simulink model "Mojtaba_simulink"  (R2022b)
settings: Solver=FixedStepAuto  StartTime=0.0  StopTime=5  FixedStep=1e-3  RelTol=1e-3
values from neighbouring files (symbols this model uses):
  Mojtaba_hand = Hand('Mojtaba_hand')    [create_Hand_Model_wt_Muscles.m]    (also in create_MSK_Mojtaba.m)
settings Model: Creator=ge26jow  LastModifiedBy=ge26jow

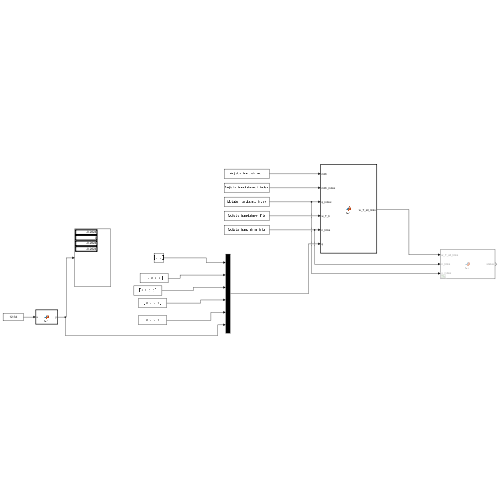
[thumbnail: Simulink's stored preview of the top-level diagram]
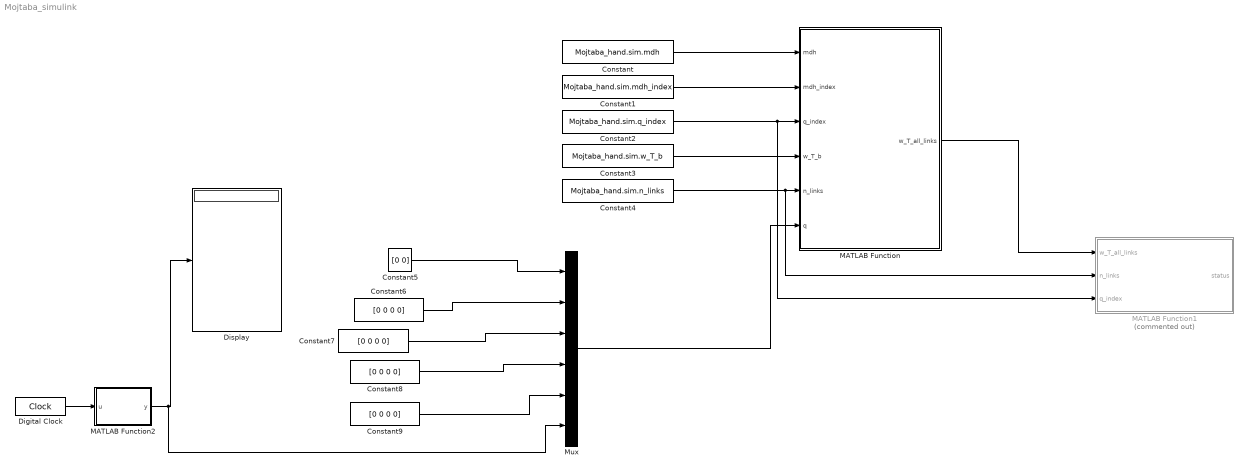
== system Mojtaba_simulink ==
  Constant : Constant  Value=Mojtaba_hand.sim.mdh
  Constant1 : Constant  Value=Mojtaba_hand.sim.mdh_index
  Constant2 : Constant  Value=Mojtaba_hand.sim.q_index
  Constant3 : Constant  Value=Mojtaba_hand.sim.w_T_b
  Constant4 : Constant  Value=Mojtaba_hand.sim.n_links
  Constant5 : Constant  Value=[0 0]
  Constant{6..9} (4 alike) : Constant  Value=[0 0 0 0]
  Digital Clock : DigitalClock  SampleTime=1e-2
  Display : Display
  MATLAB Function : MATLAB Function  TreatAsAtomicUnit=on
  MATLAB Function1 : MATLAB Function  Commented=on  TreatAsAtomicUnit=on
  MATLAB Function2 : MATLAB Function  TreatAsAtomicUnit=on
  Mux : Mux  Inputs=6
  wires:
  Constant/1 -> MATLAB Function/1(mdh)
  Constant1/1 -> MATLAB Function/2(mdh_index)
  Constant2/1 -> MATLAB Function1/3(q_index), MATLAB Function/3(q_index)
  Constant3/1 -> MATLAB Function/4(w_T_b)
  Constant4/1 -> MATLAB Function1/2(n_links), MATLAB Function/5(n_links)
  MATLAB Function/1(w_T_all_links) -> MATLAB Function1/1(w_T_all_links)
  Constant5/1 -> Mux/1
  Constant6/1 -> Mux/2
  Constant8/1 -> Mux/4
  Constant9/1 -> Mux/5
  Mux/1 -> MATLAB Function/6(q)
  MATLAB Function2/1(y) -> Mux/6, Display/1
  Digital Clock/1 -> MATLAB Function2/1(u)
  Constant7/1 -> Mux/3

== matlab function Mojtaba_simulink/MATLAB Function1 ==
  data: w_T_all_links input; status output; n_links input; q_index input
function status = fcn(w_T_all_links,n_links,q_index)
status = sim_plot_hand(w_T_all_links,n_links,q_index);

== matlab function Mojtaba_simulink/MATLAB Function ==
  data: mdh input; w_T_all_links output; mdh_index input; q_index input; w_T_b input; n_links input; q input
function w_T_all_links = fcn(mdh,mdh_index,q_index,w_T_b,n_links,q)

w_T_all_links = sim_w_T_all_links_from_q(mdh,mdh_index,q_index,w_T_b,n_links,q);

== matlab function Mojtaba_simulink/MATLAB Function2 ==
  data: u input; y output
function y = fcn(u)

y = [sin(10*u),0,sin(10*u),sin(10*u)]';
